simulink model "lab_3_task_1_simulink"  (R2025b)
settings: Solver=ode5  StartTime=0.0  StopTime=200  FixedStep=0.5  RelTol=1e-3
values from neighbouring files (symbols this model uses):
  ix = 0.070    (= 0.07)    [lab_3_task_1.m]    (also in lab_3_task_3.m = 0.025; lab_4_task_3.m; lab_5_task_1.m; lab_5_task_2.m)
  iy = 0.055    [lab_3_task_1.m]    (also in lab_3_task_3.m; lab_4_task_3.m; lab_5_task_1.m; lab_5_task_2.m)
  iz = 0.025    [lab_3_task_1.m]    (also in lab_3_task_3.m = 0.07; lab_4_task_3.m; lab_5_task_1.m; lab_5_task_2.m)
  wx0 = 0.45    [lab_3_task_1.m]    (also in lab_4_task_3.m; lab_5_task_1.m; lab_5_task_2.m = 0.2 + (2*pi - 0.2)*rand; lab_6_task_1.m = 0)
  wy0 = 0.52    [lab_3_task_1.m]    (also in lab_4_task_3.m; lab_5_task_1.m; lab_5_task_2.m = 0.1; lab_6_task_1.m = 0)
  wz0 = 0.55    [lab_3_task_1.m]    (also in lab_4_task_3.m; lab_5_task_1.m; lab_5_task_2.m = 0.1; lab_6_task_1.m = n)
settings Model: Creator=User  LastModifiedBy=User

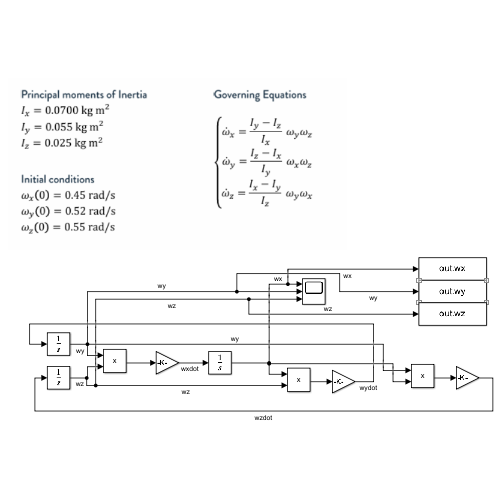
[thumbnail: Simulink's stored preview of the top-level diagram]
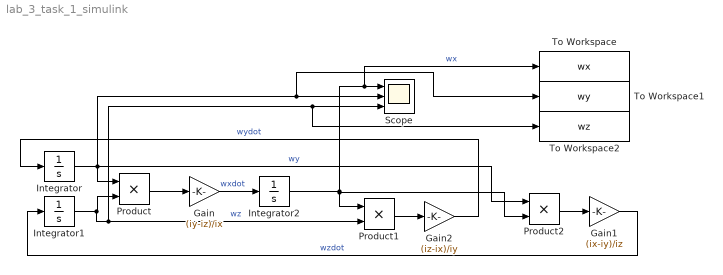
== system lab_3_task_1_simulink ==
  Gain : Gain  Gain=(iy-iz)/ix
  Gain1 : Gain  Gain=(ix-iy)/iz
  Gain2 : Gain  Gain=(iz-ix)/iy
  Integrator : Integrator  InitialCondition=wy0
  Integrator1 : Integrator  InitialCondition=wz0
  Integrator2 : Integrator  InitialCondition=wx0
  Product : Product
  Product1 : Product
  Product2 : Product
  Scope : Scope  NumInputPorts=3
  To Workspace : ToWorkspace  VariableName=wx  SaveFormat=Timeseries  SampleTime=-1
  To Workspace1 : ToWorkspace  VariableName=wy  SaveFormat=Timeseries  SampleTime=-1
  To Workspace2 : ToWorkspace  VariableName=wz  SaveFormat=Timeseries  SampleTime=-1
  wires:
  Integrator1/1 -> To Workspace2/1, Scope/3, Product1/2, Product/2  "wz"
  Integrator/1 -> To Workspace1/1, Scope/2, Product2/1, Product/1  "wy"
  Integrator2/1 -> Product2/2, Product1/1, To Workspace/1, Scope/1  "wx"
  Product1/1 -> Gain2/1
  Product/1 -> Gain/1
  Gain/1 -> Integrator2/1  "wxdot"
  Gain2/1 -> Integrator/1  "wydot"
  Product2/1 -> Gain1/1
  Gain1/1 -> Integrator1/1  "wzdot"
